simulink subsystem "Unstable_plant_model"  (R2024b)
settings: Solver=VariableStepAuto  StartTime=0.0  StopTime=10.0  RelTol=1e-3
settings Model: Creator=tshintai  LastModifiedBy=tshintai
settings SolverCC: AlgebraicLoopSolver=TrustRegion
settings OptimizationCC: ReuseModelBlockBuffer=off
settings DebuggingCC: UnconnectedInputMsg=warning  UnconnectedOutputMsg=warning  UnconnectedLineMsg=warning
settings ModelReferenceCC: EnableRefExpFcnMdlSchedulingChecks=on
settings RTWCC: GPUComputeCapability=3.5  DLArmComputeVersion=19.05

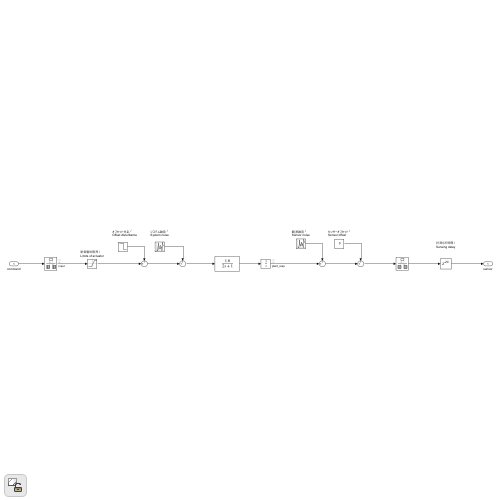
[thumbnail: Simulink's stored preview of the top-level diagram]
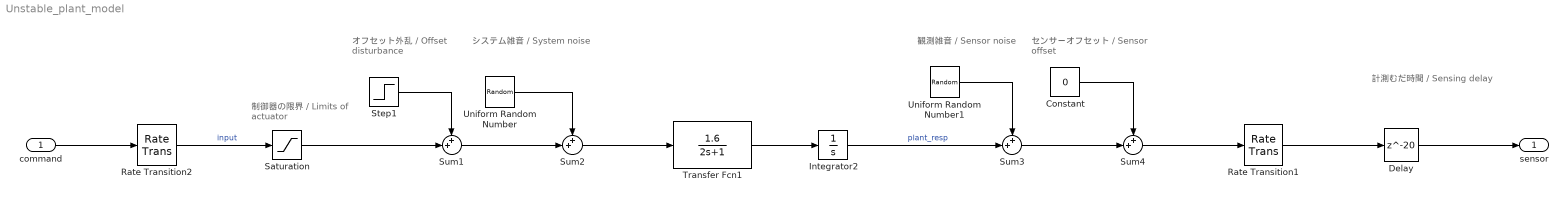
== system Unstable_plant_model ==
  note: 観測雑音 /
      | Sensor noise
  note: 制御器の限界 /
      | Limits of actuator
  note: システム雑音 /
      | System noise
  note: 計測むだ時間 /
      | Sensing delay
  note: オフセット外乱 /
      | Offset disturbance
  note: センサーオフセット /
      | Sensor offset
  command : Inport
  Constant : Constant  Value=0
  Delay : Delay  DelayLength=20
  Integrator2 : Integrator
  Rate Transition1 : RateTransition  OutPortSampleTime=TimeStep
  Rate Transition2 : RateTransition
  Saturation : Saturate  UpperLimit=0.2  LowerLimit=-0.2
  Step1 : Step  Time=20  After=-0.1  SampleTime=0
  Sum{1..4} (4 alike) : Sum  Inputs=++|
  Transfer Fcn1 : TransferFcn  Numerator=[1.6]  Denominator=[2 1]
  Uniform Random Number : UniformRandomNumber  Minimum=-0.2  Maximum=0.2  SampleTime=0
  Uniform Random Number1 : UniformRandomNumber  Minimum=-0.1  Maximum=0.1  Seed=1  SampleTime=0
  sensor : Outport
  wires:
  Step1/1 -> Sum1/1
  Uniform Random Number1/1 -> Sum3/1
  Sum4/1 -> Rate Transition1/1
  Sum2/1 -> Transfer Fcn1/1
  Rate Transition2/1 -> Saturation/1  "input"
  Uniform Random Number/1 -> Sum2/1
  Saturation/1 -> Sum1/2
  Sum1/1 -> Sum2/2
  Integrator2/1 -> Sum3/2  "plant_resp"
  Constant/1 -> Sum4/1
  Transfer Fcn1/1 -> Integrator2/1
  Sum3/1 -> Sum4/2
  Rate Transition1/1 -> Delay/1
  Delay/1 -> sensor/1
  command/1 -> Rate Transition2/1
